simulink model "practical_class_2_1b_simulink"  (R2023b)
settings: Solver=VariableStepAuto  StartTime=0.0  StopTime=45  RelTol=1e-3
undefined symbols (not defined in the file): den1, den2, num1, num2
settings Model: Creator=klysm  LastModifiedBy=klysm

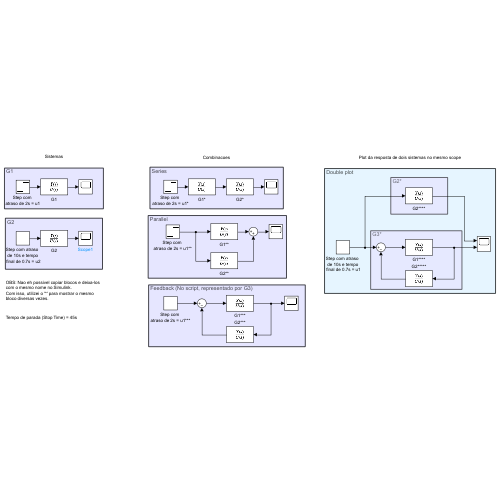
[thumbnail: Simulink's stored preview of the top-level diagram]
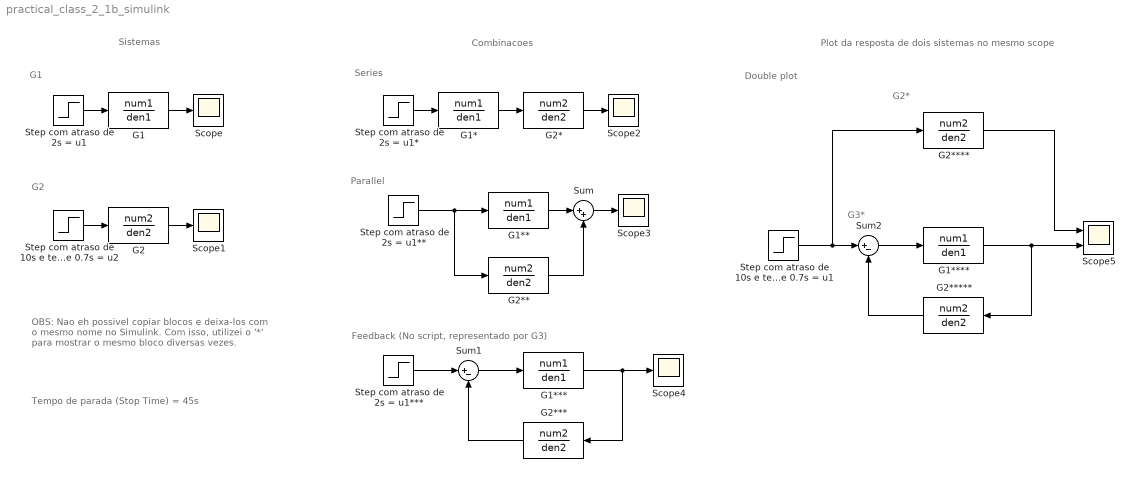
== system practical_class_2_1b_simulink ==
  note: Plot da resposta de dois sistemas no mesmo scope
  note: Double plot
  note: G2*
  note: G3*
  note: Tempo de parada (Stop Time) = 45s
  note: OBS: Nao eh possivel copiar blocos e deixa-los com o mesmo nome no Simulink.
      | Com isso, utilizei o '*' para mostrar o mesmo bloco diversas vezes.
  note: Feedback (No script, representado por G3)
  note: Combinacoes
  note: Sistemas
  note: Parallel
  note: Series
  note: G2
  note: G1
  G1 : TransferFcn  Numerator=num1  Denominator=den1
  G1* : TransferFcn  Numerator=num1  Denominator=den1
  G1** : TransferFcn  Numerator=num1  Denominator=den1
  G1*** : TransferFcn  Numerator=num1  Denominator=den1
  G1**** : TransferFcn  Numerator=num1  Denominator=den1
  G2 : TransferFcn  Numerator=num2  Denominator=den2
  G2* : TransferFcn  Numerator=num2  Denominator=den2
  G2** : TransferFcn  Numerator=num2  Denominator=den2
  G2*** : TransferFcn  Numerator=num2  Denominator=den2
  G2**** : TransferFcn  Numerator=num2  Denominator=den2
  G2***** : TransferFcn  Numerator=num2  Denominator=den2
  Scope{,1..4} (5 alike) : Scope
  Scope5 : Scope  NumInputPorts=2
  Step com atraso de 2s = u1 : Step  Time=2  SampleTime=0
  Step com atraso de 2s = u1* : Step  Time=2  SampleTime=0
  Step com atraso de 2s = u1** : Step  Time=2  SampleTime=0
  Step com atraso de 2s = u1*** : Step  Time=2  SampleTime=0
  Step com atraso de 10s e tempo final de 0.7s = u1 : Step  SampleTime=0
  Step com atraso de 10s e tempo final de 0.7s = u2 : Step  SampleTime=0
  Sum : Sum  Inputs=|++
  Sum1 : Sum  Inputs=|+-
  Sum2 : Sum  Inputs=|+-
  wires:
  G1/1 -> Scope/1
  Step com atraso de 2s = u1/1 -> G1/1
  Step com atraso de 10s e tempo final de 0.7s = u2/1 -> G2/1
  G2/1 -> Scope1/1
  G1*/1 -> G2*/1
  Step com atraso de 2s = u1*/1 -> G1*/1
  G2*/1 -> Scope2/1
  G1**/1 -> Sum/1
  G2**/1 -> Sum/2
  Sum/1 -> Scope3/1
  Step com atraso de 2s = u1**/1 -> G2**/1, G1**/1
  G1***/1 -> G2***/1, Scope4/1
  Step com atraso de 2s = u1***/1 -> Sum1/1
  Sum1/1 -> G1***/1
  G2***/1 -> Sum1/2
  Sum2/1 -> G1****/1
  G2*****/1 -> Sum2/2
  G1****/1 -> G2*****/1, Scope5/2
  G2****/1 -> Scope5/1
  Step com atraso de 10s e tempo final de 0.7s = u1/1 -> G2****/1, Sum2/1
